simulink library "dcpctrl"  (R2016a)
settings: Solver=ode45  StartTime=0.0  StopTime=10.0  RelTol=1e-3
values from neighbouring files (symbols this model uses):
  robot = struct('Name', 'DCP_V2')    [config_dcpv2.m]
undefined symbols (not defined in the file or in its folder): Humusoft, MF644, Standard_Devices, UDP_Protocol
libraries: sldrtlib x6, simulink x2, dspsigops x1
settings Model: Creator=julianleland  LastModifiedBy=julianleland
settings DataIOCC: LimitDataPoints=on
settings DebuggingCC: AllowSymbolicDim=off

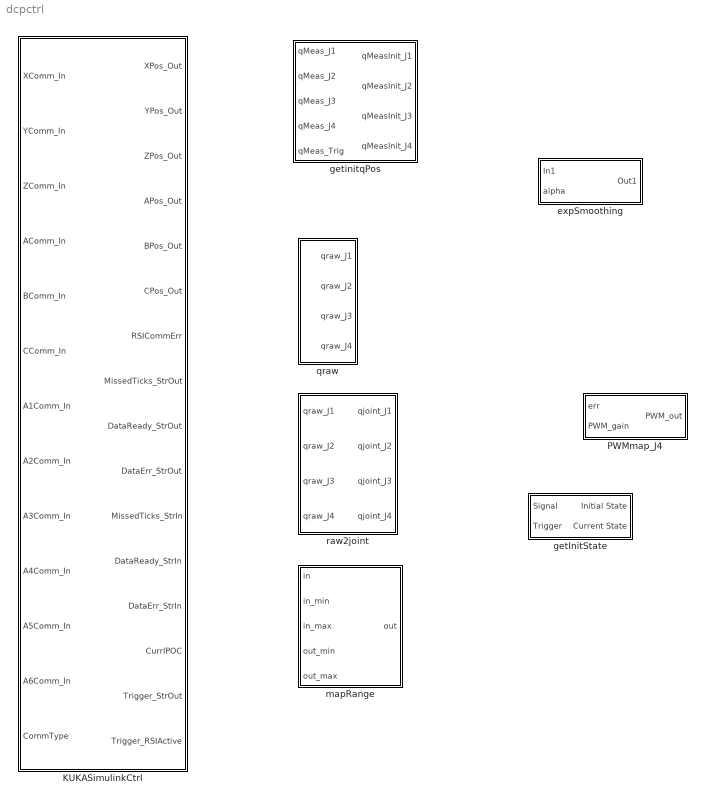
== system dcpctrl ==
  KUKASimulinkCtrl : Subsystem
  PWMmap_J4 : Subsystem
  expSmoothing : Subsystem
  getInitState : Subsystem
  getinitqPos : Subsystem
  "mapRange " : MATLAB Function  TreatAsAtomicUnit=on
  qraw : Subsystem
  raw2joint : Subsystem

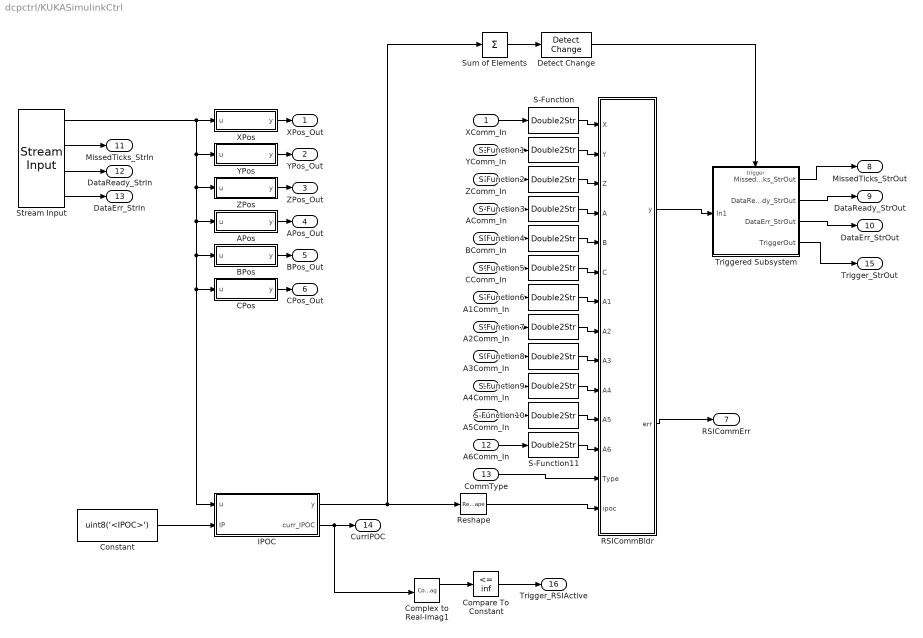
== system dcpctrl/KUKASimulinkCtrl ==
  XComm_In : Inport
  YComm_In : Inport  Port=2
  ZComm_In : Inport  Port=3
  AComm_In : Inport  Port=4
  BComm_In : Inport  Port=5
  CComm_In : Inport  Port=6
  A1Comm_In : Inport  Port=7
  A2Comm_In : Inport  Port=8
  A3Comm_In : Inport  Port=9
  A4Comm_In : Inport  Port=10
  A5Comm_In : Inport  Port=11
  A6Comm_In : Inport  Port=12
  CommType : Inport  Port=13
  APos : MATLAB Function  TreatAsAtomicUnit=on
  BPos : MATLAB Function  TreatAsAtomicUnit=on
  CPos : MATLAB Function  TreatAsAtomicUnit=on
  Compare To Constant : simulink/Logic and Bit Operations/Compare To Constant  relop=<=  const=inf  OutDataTypeStr=boolean
  Complex to Real-Imag1 : ComplexToRealImag
  Constant : Constant  Value=uint8('<IPOC>')
  Detect Change : simulink/Logic and Bit Operations/Detect Change  vinit=0  OutDataTypeStr=boolean
  IPOC : MATLAB Function  TreatAsAtomicUnit=on
  RSICommBldr : MATLAB Function  TreatAsAtomicUnit=on
  Reshape : Reshape
  S-Function{,1..11} (12 alike) : S-Function  FunctionName=Double2Str  SFunctionDeploymentMode=off  EnableBusSupport=off
  Stream Input : sldrtlib/Stream Input  SampleTime=-1  MaxMissedTicks=10  ShowMissedTicks=on  YieldWhenWaiting=on  DrvName=Standard_Devices/UDP_Protocol  DrvAddress=27277  DrvOptions=[174338148 53453]  DataTypes='238*uint16'  FormatString=repmat('%c',1,238)  Terminator='/Rob>'  ShowReady=on  ShowError=on
      settings: AttributesFormatString=Standard Devices\nUDP Protocol [6A8Dh]
  Sum of Elements : Sum  Inputs=+  CollapseMode=Specified dimension  CollapseDim=2
  Triggered Subsystem : Subsystem  TreatAsAtomicUnit=on
  XPos : MATLAB Function  TreatAsAtomicUnit=on
  YPos : MATLAB Function  TreatAsAtomicUnit=on
  ZPos : MATLAB Function  TreatAsAtomicUnit=on
  XPos_Out : Outport
  YPos_Out : Outport  Port=2
  ZPos_Out : Outport  Port=3
  APos_Out : Outport  Port=4
  BPos_Out : Outport  Port=5
  CPos_Out : Outport  Port=6
  RSICommErr : Outport  Port=7
  MissedTicks_StrOut : Outport  Port=8
  DataReady_StrOut : Outport  Port=9
  DataErr_StrOut : Outport  Port=10
  MissedTicks_StrIn : Outport  Port=11
  DataReady_StrIn : Outport  Port=12
  DataErr_StrIn : Outport  Port=13
  CurrIPOC : Outport  Port=14
  Trigger_StrOut : Outport  Port=15
  Trigger_RSIActive : Outport  Port=16
  wires:
  YComm_In/1 -> S-Function1/1
  BPos/1(y) -> BPos_Out/1
  CComm_In/1 -> S-Function5/1
  ZComm_In/1 -> S-Function2/1
  AComm_In/1 -> S-Function3/1
  BComm_In/1 -> S-Function4/1
  A6Comm_In/1 -> S-Function11/1
  RSICommBldr/2(err) -> RSICommErr/1
  A5Comm_In/1 -> S-Function10/1
  XPos/1(y) -> XPos_Out/1
  A2Comm_In/1 -> S-Function7/1
  A4Comm_In/1 -> S-Function9/1
  APos/1(y) -> APos_Out/1
  A3Comm_In/1 -> S-Function8/1
  YPos/1(y) -> YPos_Out/1
  A1Comm_In/1 -> S-Function6/1
  ZPos/1(y) -> ZPos_Out/1
  XComm_In/1 -> S-Function/1
  CPos/1(y) -> CPos_Out/1
  Stream Input/3 -> DataReady_StrIn/1
  S-Function/1 -> RSICommBldr/1(X)
  Stream Input/2 -> MissedTicks_StrIn/1
  Stream Input/1 -> IPOC/1(u), CPos/1(u), BPos/1(u), APos/1(u), ZPos/1(u), YPos/1(u), XPos/1(u)
  RSICommBldr/1(y) -> Triggered Subsystem/1(In1)
  IPOC/1(y) -> Sum of Elements/1, Reshape/1
  Constant/1 -> IPOC/2(IP)
  S-Function1/1 -> RSICommBldr/2(Y)
  S-Function2/1 -> RSICommBldr/3(Z)
  S-Function3/1 -> RSICommBldr/4(A)
  S-Function4/1 -> RSICommBldr/5(B)
  S-Function5/1 -> RSICommBldr/6(C)
  S-Function6/1 -> RSICommBldr/7(A1)
  S-Function7/1 -> RSICommBldr/8(A2)
  S-Function8/1 -> RSICommBldr/9(A3)
  S-Function9/1 -> RSICommBldr/10(A4)
  S-Function10/1 -> RSICommBldr/11(A5)
  S-Function11/1 -> RSICommBldr/12(A6)
  Triggered Subsystem/1(MissedTicks_StrOut) -> MissedTicks_StrOut/1
  Triggered Subsystem/2(DataReady_StrOut) -> DataReady_StrOut/1
  Triggered Subsystem/3(DataErr_StrOut) -> DataErr_StrOut/1
  Stream Input/4 -> DataErr_StrIn/1
  IPOC/2(curr_IPOC) -> Complex to Real-Imag1/1, CurrIPOC/1
  Reshape/1 -> RSICommBldr/14(ipoc)
  CommType/1 -> RSICommBldr/13(Type)
  Triggered Subsystem/4(TriggerOut) -> Trigger_StrOut/1
  Detect Change/1 -> Triggered Subsystem/Trigger
  Sum of Elements/1 -> Detect Change/1
  Compare To Constant/1 -> Trigger_RSIActive/1
  Complex to Real-Imag1/1 -> Compare To Constant/1

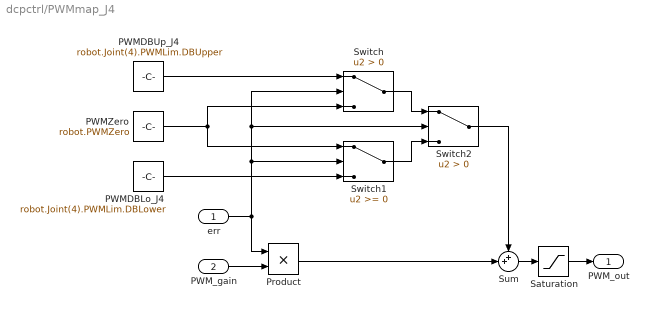
== system dcpctrl/PWMmap_J4 ==
  err : Inport
  "PWM_gain " : Inport  Port=2
  PWMDBLo_J4 : Constant  Value=robot.Joint(4).PWMLim.DBLower
  PWMDBUp_J4 : Constant  Value=robot.Joint(4).PWMLim.DBUpper
  PWMZero : Constant  Value=robot.PWMZero
  Product : Product
  Saturation : Saturate  UpperLimit=robot.Joint(4).PWMLim.Max  LowerLimit=robot.Joint(4).PWMLim.Min
  Sum : Sum  Inputs=++|
  Switch : Switch  Criteria=u2 > Threshold
  Switch1 : Switch
  Switch2 : Switch  Criteria=u2 > Threshold
  PWM_out : Outport
  wires:
  Sum/1 -> Saturation/1
  "PWM_gain "/1 -> Product/2
  err/1 -> Product/1, Switch1/2, Switch2/2, Switch/2
  Product/1 -> Sum/2
  PWMDBUp_J4/1 -> Switch/1
  Saturation/1 -> PWM_out/1
  PWMDBLo_J4/1 -> Switch1/3
  PWMZero/1 -> Switch1/1, Switch/3
  Switch1/1 -> Switch2/3
  Switch/1 -> Switch2/1
  Switch2/1 -> Sum/1

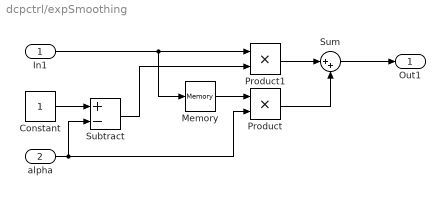
== system dcpctrl/expSmoothing ==
  In1 : Inport
  alpha : Inport  Port=2
  Constant : Constant
  Memory : Memory
  Product : Product
  Product1 : Product
  Subtract : Sum  Inputs=+-
  Sum : Sum  Inputs=|++
  Out1 : Outport
  wires:
  In1/1 -> Product1/1, Memory/1
  Memory/1 -> Product/1
  alpha/1 -> Subtract/2, Product/2
  Product1/1 -> Sum/1
  Product/1 -> Sum/2
  Sum/1 -> Out1/1
  Constant/1 -> Subtract/1
  Subtract/1 -> Product1/2

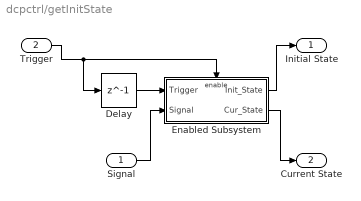
== system dcpctrl/getInitState ==
  Signal : Inport
  Trigger : Inport  Port=2
  Delay : Delay  DelayLength=1  InitialCondition=0
  Enabled Subsystem : Subsystem  TreatAsAtomicUnit=on
  Initial State : Outport
  Current State : Outport  Port=2
  wires:
  Delay/1 -> Enabled Subsystem/1(Trigger)
  Trigger/1 -> Enabled Subsystem/Enable, Delay/1
  Enabled Subsystem/2(Cur_State) -> Current State/1
  Enabled Subsystem/1(Init_State) -> Initial State/1
  Signal/1 -> Enabled Subsystem/2(Signal)

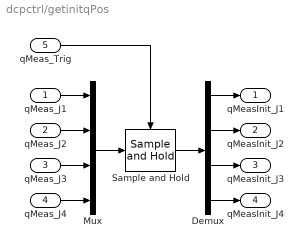
== system dcpctrl/getinitqPos ==
  qMeas_J1 : Inport
  qMeas_J2 : Inport  Port=2
  qMeas_J3 : Inport  Port=3
  qMeas_J4 : Inport  Port=4
  qMeas_Trig : Inport  Port=5
  Demux : Demux
  Mux : Mux
  Sample and Hold : dspsigops/Sample and Hold  trig=Rising edge  initCond=0  latchinput=off
  qMeasInit_J1 : Outport
  qMeasInit_J2 : Outport  Port=2
  qMeasInit_J3 : Outport  Port=3
  qMeasInit_J4 : Outport  Port=4
  wires:
  qMeas_Trig/1 -> Sample and Hold/Trigger
  qMeas_J4/1 -> Mux/4
  qMeas_J3/1 -> Mux/3
  qMeas_J2/1 -> Mux/2
  qMeas_J1/1 -> Mux/1
  Demux/2 -> qMeasInit_J2/1
  Demux/3 -> qMeasInit_J3/1
  Demux/4 -> qMeasInit_J4/1
  Demux/1 -> qMeasInit_J1/1
  Sample and Hold/1 -> Demux/1
  Mux/1 -> Sample and Hold/1

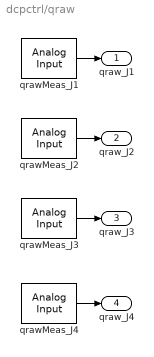
== system dcpctrl/qraw ==
  qrawMeas_J1 : sldrtlib/Analog Input  SampleTime=-1  MaxMissedTicks=10  ShowMissedTicks=off  YieldWhenWaiting=off  DrvName=Humusoft/MF644  DrvAddress=4294967295  DrvOptions=585  Channels=2  RangeMode=1  VoltRange=1  DataType=1
      settings: AttributesFormatString=Humusoft\nMF644 [auto]
  qrawMeas_J2 : sldrtlib/Analog Input  SampleTime=-1  MaxMissedTicks=10  ShowMissedTicks=off  YieldWhenWaiting=off  DrvName=Humusoft/MF644  DrvAddress=4294967295  DrvOptions=585  Channels=3  RangeMode=1  VoltRange=1  DataType=1
      settings: AttributesFormatString=Humusoft\nMF644 [auto]
  qrawMeas_J3 : sldrtlib/Analog Input  SampleTime=-1  MaxMissedTicks=10  ShowMissedTicks=off  YieldWhenWaiting=off  DrvName=Humusoft/MF644  DrvAddress=4294967295  DrvOptions=585  Channels=4  RangeMode=1  VoltRange=1  DataType=1
      settings: AttributesFormatString=Humusoft\nMF644 [auto]
  qrawMeas_J4 : sldrtlib/Analog Input  SampleTime=-1  MaxMissedTicks=10  ShowMissedTicks=off  YieldWhenWaiting=off  DrvName=Humusoft/MF644  DrvAddress=4294967295  DrvOptions=585  Channels=5  RangeMode=1  VoltRange=1  DataType=1
      settings: AttributesFormatString=Humusoft\nMF644 [auto]
  qraw_J1 : Outport
  qraw_J2 : Outport  Port=2
  qraw_J3 : Outport  Port=3
  qraw_J4 : Outport  Port=4
  wires:
  qrawMeas_J4/1 -> qraw_J4/1
  qrawMeas_J1/1 -> qraw_J1/1
  qrawMeas_J2/1 -> qraw_J2/1
  qrawMeas_J3/1 -> qraw_J3/1

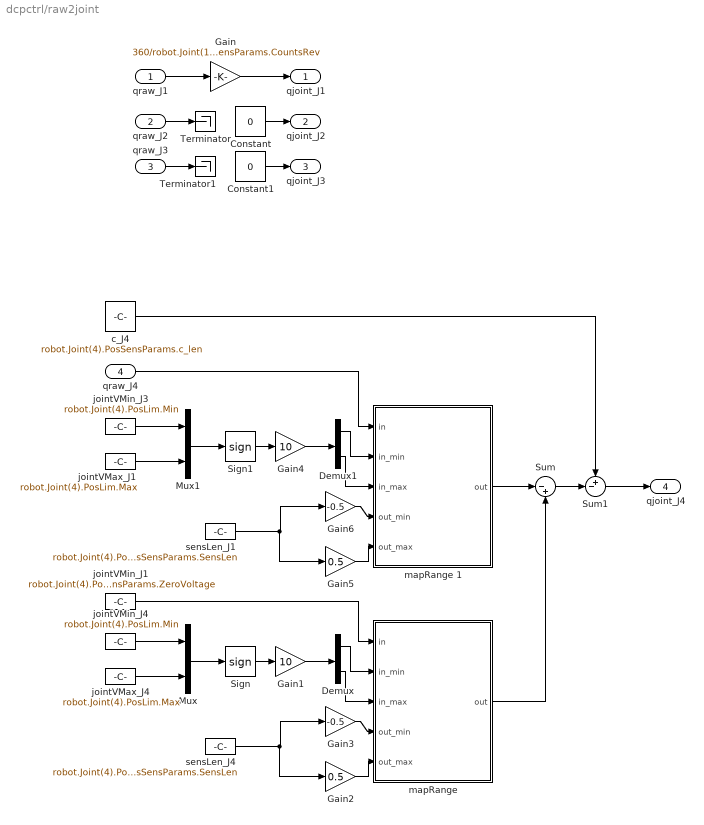
== system dcpctrl/raw2joint ==
  qraw_J1 : Inport
  qraw_J2 : Inport  Port=2
  qraw_J3 : Inport  Port=3
  qraw_J4 : Inport  Port=4
  Constant : Constant  Value=0
  Constant1 : Constant  Value=0
  Demux : Demux  Outputs=2
  Demux1 : Demux  Outputs=2
  Gain : Gain  Gain=360/robot.Joint(1).PosSensParams.CountsRev
  Gain1 : Gain  Gain=10
  Gain2 : Gain  Gain=0.5
  Gain3 : Gain  Gain=-0.5
  Gain4 : Gain  Gain=10
  Gain5 : Gain  Gain=0.5
  Gain6 : Gain  Gain=-0.5
  Mux : Mux  Inputs=2
  Mux1 : Mux  Inputs=2
  Sign : Signum
  Sign1 : Signum
  Sum : Sum  Inputs=|-+
  Sum1 : Sum  Inputs=+-|
  Terminator : Terminator
  Terminator1 : Terminator
  c_J4 : Constant  Value=robot.Joint(4).PosSensParams.c_len
  jointVMax_J1 : Constant  Value=robot.Joint(4).PosLim.Max
  jointVMax_J4 : Constant  Value=robot.Joint(4).PosLim.Max
  jointVMin_J1 : Constant  Value=robot.Joint(4).PosSensParams.ZeroVoltage
  jointVMin_J3 : Constant  Value=robot.Joint(4).PosLim.Min
  jointVMin_J4 : Constant  Value=robot.Joint(4).PosLim.Min
  "mapRange " : MATLAB Function  TreatAsAtomicUnit=on
  mapRange 1 : MATLAB Function  TreatAsAtomicUnit=on
  sensLen_J1 : Constant  Value=robot.Joint(4).PosSensParams.SensLen
  sensLen_J4 : Constant  Value=robot.Joint(4).PosSensParams.SensLen
  qjoint_J1 : Outport
  qjoint_J2 : Outport  Port=2
  qjoint_J3 : Outport  Port=3
  qjoint_J4 : Outport  Port=4
  wires:
  qraw_J1/1 -> Gain/1
  qraw_J2/1 -> Terminator/1
  qraw_J3/1 -> Terminator1/1
  Gain/1 -> qjoint_J1/1
  Mux/1 -> Sign/1
  Sign/1 -> Gain1/1
  Gain2/1 -> "mapRange "/5(out_max)
  Gain3/1 -> "mapRange "/4(out_min)
  sensLen_J4/1 -> Gain2/1, Gain3/1
  Gain1/1 -> Demux/1
  jointVMin_J4/1 -> Mux/1
  jointVMax_J4/1 -> Mux/2
  Demux/1 -> "mapRange "/2(in_min)
  Demux/2 -> "mapRange "/3(in_max)
  jointVMin_J1/1 -> "mapRange "/1(in)
  Mux1/1 -> Sign1/1
  Sign1/1 -> Gain4/1
  Gain5/1 -> mapRange 1/5(out_max)
  Gain6/1 -> mapRange 1/4(out_min)
  sensLen_J1/1 -> Gain5/1, Gain6/1
  Gain4/1 -> Demux1/1
  jointVMin_J3/1 -> Mux1/1
  jointVMax_J1/1 -> Mux1/2
  Demux1/1 -> mapRange 1/2(in_min)
  Demux1/2 -> mapRange 1/3(in_max)
  qraw_J4/1 -> mapRange 1/1(in)
  mapRange 1/1(out) -> Sum/1
  "mapRange "/1(out) -> Sum/2
  Sum/1 -> Sum1/2
  c_J4/1 -> Sum1/1
  Sum1/1 -> qjoint_J4/1
  Constant/1 -> qjoint_J2/1
  Constant1/1 -> qjoint_J3/1

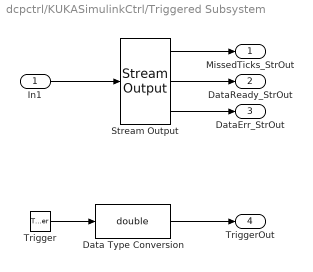
== system dcpctrl/KUKASimulinkCtrl/Triggered Subsystem ==
  In1 : Inport
  Trigger : TriggerPort  VariantControl=Variant  ShowOutputPort=on
  Data Type Conversion : DataTypeConversion  OutDataTypeStr=double
  Stream Output : sldrtlib/Stream Output  SampleTime=inf  MaxMissedTicks=10  ShowMissedTicks=on  YieldWhenWaiting=off  DrvName=Standard_Devices/UDP_Protocol  DrvAddress=27277  DrvOptions=[174338148 53453]  PortSizes=279  FormatString=repmat('%c',1,279)  ShowReady=on  ShowError=on  InitialValue=[]  FinalValue=[]
      settings: AttributesFormatString=Standard Devices\nUDP Protocol [6A8Dh]
  MissedTicks_StrOut : Outport
  DataReady_StrOut : Outport  Port=2
  DataErr_StrOut : Outport  Port=3
  TriggerOut : Outport  Port=4
  wires:
  Stream Output/1 -> MissedTicks_StrOut/1
  Stream Output/2 -> DataReady_StrOut/1
  Stream Output/3 -> DataErr_StrOut/1
  In1/1 -> Stream Output/1
  Data Type Conversion/1 -> TriggerOut/1
  Trigger/1 -> Data Type Conversion/1

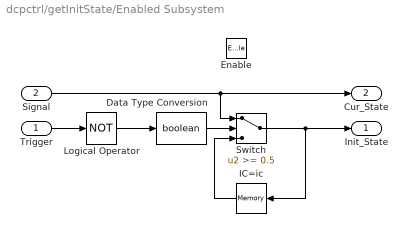
== system dcpctrl/getInitState/Enabled Subsystem ==
  Trigger : Inport
  Signal : Inport  Port=2
  Enable : EnablePort  StatesWhenEnabling=reset
  Data Type Conversion : DataTypeConversion  OutDataTypeStr=boolean
  IC=ic : Memory  LinearizeAsDelay=on
  Logical Operator : Logic  Operator=NOT  AllPortsSameDT=off  OutDataTypeStr=boolean
  Switch : Switch  Threshold=0.5  SaturateOnIntegerOverflow=on  InputSameDT=on
  Init_State : Outport
  Cur_State : Outport  Port=2
  wires:
  Signal/1 -> Switch/1, Cur_State/1
  Logical Operator/1 -> Data Type Conversion/1
  IC=ic/1 -> Switch/3
  Switch/1 -> Init_State/1, IC=ic/1
  Data Type Conversion/1 -> Switch/2
  Trigger/1 -> Logical Operator/1

== matlab function dcpctrl/KUKASimulinkCtrl/XPos ==
  data: u input; y output
function y = fcn(u)
%#codegen

% Convert input into characters.
string = char(u);

% Locate start of X and Y strings
indx_X = strfind(string','X=');
indx_Y = strfind(string','Y=');

% Once X and Y strings have been located, grab the intervening characters
% (the X position). Otherwise, set to 0.
if ~isempty(indx_X)
    str_X = string((indx_X(1)+3):(indx_Y(1)-3));
    doub_X = str2double(str_X);
    y = doub_X;
else
    y = 0.0;
% TODO: Is this safe? Probably - if we're in abs mode and we command zero
% from some far distance away, it will cause a fault.
end

== matlab function dcpctrl/KUKASimulinkCtrl/RSICommBldr ==
  data: X input; Y input; Z input; A input; B input; C input; A1 input; A2 input; A3 input; A4 input; A5 input; A6 input; Type input; y output; ipoc input; err output
function [y, err] = fcn(X,Y,Z,A,B,C,A1,A2,A3,A4,A5,A6,Type,ipoc)
%#codegen

err = 0; % Default: define no error state.

%{
% Check whether we're inputting a RKorr or AKorr
switch Type
    case 82 % Either 'R' or 'r' passed in as uint8 - 82 or 114
        s1 = uint8('<Sen Type="ImFree"><RKorr ');
        s2 = uint8('X="');
        s3 = uint8('" Y="');
        s4 = uint8('" Z="');
        s5 = uint8('" A="');
        s6 = uint8('" B="');
        s7 = uint8('" C="');
        s8 = uint8('" /><IPOC>');
        s9 = uint8('</IPOC></Sen>');
        y = [s1 s2 X' s3 Y' s4 Z' s5 A' s6 B' s7 C' s8 ipoc' s9]
    case 65 % Either 'A' or 'a' passed in as uint8 - 65 or 97
        y = uint8('<Sen Type="ImFree"><RKorr '); % DUMMY - write correct string for analog input here instead
    otherwise
        y = uint8(''); % Send empty string so that KUKA gets upset
        err = 1; % Set error flag to 1
%}

crlf = [char(13) char(10)]; % Carriage return plus line feed
s1 = uint8(['<Sen Type="ImFree">' crlf]);
s1p1 = uint8(['<EStr></EStr>' crlf]);
s1p2 = uint8(['<Tech T21="1.09" T22="2.08" T23="3.07" T24="4.06" T25="5.05" T26="6.04" T27="7.03" T28="8.02" T29="9.01" T210="10.00" />' crlf]);
s1p3 = uint8('<RKorr ');
s2 = uint8('X="');
s3 = uint8('" Y="');
s4 = uint8('" Z="');
s5 = uint8('" A="');
s6 = uint8('" B="');
s7 = uint8('" C="');
s8 = uint8(['" />' crlf]);
s9 = uint8(['<DiO>125</DiO>' crlf]);
s10 = uint8('<IPOC>');
s11 = uint8(['</IPOC>' crlf]);
s12 = uint8('</Sen>');
%{
s8 = uint8('" /><IPOC>');
s9 = uint8('</IPOC><DiO>125</DiO></Sen>');
%}
y = [s1 s1p1 s1p2 s1p3 s2 X' s3 Y' s4 Z' s5 A' s6 B' s7 C' s8 s9 s10 ipoc' s11 s12];

end

== matlab function dcpctrl/KUKASimulinkCtrl/YPos ==
  data: u input; y output
function y = fcn(u)
%#codegen

% Convert input into characters.
string = char(u);

% Locate start of X and Y strings
indx_Y = strfind(string','Y=');
indx_Z = strfind(string','Z=');

% Once X and Y strings have been located, grab the intervening characters
% (the X position). Otherwise, set to 0.
if ~isempty(indx_Y)
    str_Y = string((indx_Y(1)+3):(indx_Z(1)-3));
    doub_Y = str2double(str_Y);
    y = doub_Y;
else
    y = 0.0;
% TODO: Is this safe? Probably - if we're in abs mode and we command zero
% from some far distance away, it will cause a fault.
end

== matlab function dcpctrl/KUKASimulinkCtrl/ZPos ==
  data: u input; y output
function y = fcn(u)
%#codegen

% Convert input into characters.
string = char(u);

% Locate start of X and Y strings
indx_Z = strfind(string','Z=');
indx_A = strfind(string','A=');

% Once X and Y strings have been located, grab the intervening characters
% (the X position). Otherwise, set to 0.
if ~isempty(indx_Z)
    str_Z = string((indx_Z(1)+3):(indx_A(1)-3));
    doub_Z = str2double(str_Z);
    y = doub_Z;
else
    y = 0.0;
% TODO: Is this safe? Probably - if we're in abs mode and we command zero
% from some far distance away, it will cause a fault.
end

== matlab function dcpctrl/KUKASimulinkCtrl/APos ==
  data: u input; y output
function y = fcn(u)
%#codegen

% Convert input into characters.
string = char(u);

% Locate start of X and Y strings
indx_A = strfind(string','A=');
indx_B = strfind(string','B=');

% Once X and Y strings have been located, grab the intervening characters
% (the X position). Otherwise, set to 0.
if ~isempty(indx_A)
    str_A = string((indx_A(1)+3):(indx_B(1)-3));
    doub_A = str2double(str_A);
    y = doub_A;
else
    y = 0.0;
% TODO: Is this safe? Probably - if we're in abs mode and we command zero
% from some far distance away, it will cause a fault.
end

== matlab function dcpctrl/KUKASimulinkCtrl/BPos ==
  data: u input; y output
function y = fcn(u)
%#codegen

% Convert input into characters.
string = char(u);

% Locate start of X and Y strings
indx_B = strfind(string','B=');
indx_C = strfind(string','C=');

% Once X and Y strings have been located, grab the intervening characters
% (the X position). Otherwise, set to 0.
if ~isempty(indx_B)
    str_B = string((indx_B(1)+3):(indx_C(1)-3));
    doub_B = str2double(str_B);
    y = doub_B;
else
    y = 0.0;
% TODO: Is this safe? Probably - if we're in abs mode and we command zero
% from some far distance away, it will cause a fault.
end

== matlab function dcpctrl/KUKASimulinkCtrl/CPos ==
  data: u input; y output
function y = fcn(u)
%#codegen

% Convert input into characters.
string = char(u);

% Locate start of X and Y strings
indx_C = strfind(string','C=');
indx_RSol = strfind(string','/><AIPos');

% Once X and Y strings have been located, grab the intervening characters
% (the X position). Otherwise, set to 0.
if ~isempty(indx_C)
    str_C = string((indx_C(1)+3):(indx_RSol(1)-3));
    doub_C = str2double(str_C);
    y = doub_C;
else
    y = 0.0;
% TODO: Is this safe? Probably - if we're in abs mode and we command zero
% from some far distance away, it will cause a fault.
end

== matlab function dcpctrl/KUKASimulinkCtrl/IPOC ==
  data: u input; y output; IP input; curr_IPOC output
function [y, curr_IPOC] = fcn(u, IP)
%#codegen

pos = 1;
pos_end = 2;
startStrLen = 6; % Length of IPOC start string. Hard-coded for speed
lenU = length(u);
%disp(['Reading input:' u']);

for i = 1:length(u)-startStrLen
    % Compare every set of 6 elements to IPOC start string. If their sum is
    % 6, we've found the start of the string.
    if (sum(u(i:i+(startStrLen-1)) == IP) == 6)
        pos = i+startStrLen;
    end
end

for i = pos:lenU
    if (u(i) == 60) % Search for next '<' character after IPOC
        pos_end = i-1;
        break; % Need to stop searching after we've found the end of the string
    end
end

% Pad IPOC with zeroes

ipocval = u(pos:pos_end);
ipoclen = length(ipocval);

ipoctemp = ones(1,8)*48;% zeros(1,10); % We may need to change this to ones(1,10)*48 if KUKA is looking for IPOC to be padded with zeroes before start.
for n = 7:-1:7-length(ipocval)+1
    ipoctemp(n) = ipocval(end-(7-n));
end

curr_IPOC = str2double(char(ipocval));
y = uint8(ipoctemp(1:7));

== matlab function dcpctrl/mapRange  ==
  data: in input; out output; in_min input; in_max input; out_min input; out_max input
function out = mapRange(in, in_min, in_max, out_min, out_max )
%MAPRANGE Map value from one range to a second range.

% [ out_value ] = mapRange(x, in_min, in_max, out_min, out_max )
%   Julian Leland, MIT Media Lab, 2016-06-07
%   Exact knockoff of Arduino map function - see here for details: 
%   https://www.arduino.cc/en/Reference/Map
%   INPUTS:
%   x - input value to be mapped. May be a vector.
%   in_min - minumum value in range that is being mapped from
%   in_max - maximum value in range that is being mapped from
%   out_min - minimum value in range that is being mapped to
%   out_max - maximum value in range that is being mapped to
%
%   Example usage:
%   foo = [100;5;3]
%   bar = mapRange(foo,0,100,500,1000)
%   bar = [1000;525;515]

out = ((in-in_min).*(out_max-out_min))./(in_max-in_min)+out_min;

end

== matlab function dcpctrl/raw2joint/mapRange  ==
  data: in input; out output; in_min input; in_max input; out_min input; out_max input
function out = mapRange(in, in_min, in_max, out_min, out_max )
%MAPRANGE Map value from one range to a second range.

% [ out_value ] = mapRange(x, in_min, in_max, out_min, out_max )
%   Julian Leland, MIT Media Lab, 2016-06-07
%   Exact knockoff of Arduino map function - see here for details: 
%   https://www.arduino.cc/en/Reference/Map
%   INPUTS:
%   x - input value to be mapped. May be a vector.
%   in_min - minumum value in range that is being mapped from
%   in_max - maximum value in range that is being mapped from
%   out_min - minimum value in range that is being mapped to
%   out_max - maximum value in range that is being mapped to
%
%   Example usage:
%   foo = [100;5;3]
%   bar = mapRange(foo,0,100,500,1000)
%   bar = [1000;525;515]

out = ((in-in_min).*(out_max-out_min))./(in_max-in_min)+out_min;

end

== matlab function dcpctrl/raw2joint/mapRange 1 ==
  data: in input; out output; in_min input; in_max input; out_min input; out_max input
function out = mapRange(in, in_min, in_max, out_min, out_max )
%MAPRANGE Map value from one range to a second range.

% [ out_value ] = mapRange(x, in_min, in_max, out_min, out_max )
%   Julian Leland, MIT Media Lab, 2016-06-07
%   Exact knockoff of Arduino map function - see here for details: 
%   https://www.arduino.cc/en/Reference/Map
%   INPUTS:
%   x - input value to be mapped. May be a vector.
%   in_min - minumum value in range that is being mapped from
%   in_max - maximum value in range that is being mapped from
%   out_min - minimum value in range that is being mapped to
%   out_max - maximum value in range that is being mapped to
%
%   Example usage:
%   foo = [100;5;3]
%   bar = mapRange(foo,0,100,500,1000)
%   bar = [1000;525;515]

out = ((in-in_min).*(out_max-out_min))./(in_max-in_min)+out_min;

end
